simulink model "Ex_2"  (R2016b)
settings: Solver=ode3  StartTime=0.0  StopTime=10.0  RelTol=1e-3
libraries: Rayannik x3
settings Model: ExtModeTrigDuration=1000001  Creator=Alireza7  LastModifiedBy=Alireza7
settings RTWCC: SystemTargetFile=sldrt.tlc  TemplateMakefile=sldrt.tmf  Description=Simulink Desktop Real-Time  RTWCompilerOptimization=on
settings CodeAppCC: MaxIdLength=95
settings SimulinkDesktopRealTimeCC: TargetPreCompLibLocation=C:\Program Files\MATLAB\R2016b\toolbox\sldrt\lib\win64  SupportVariableSizeSignals=off

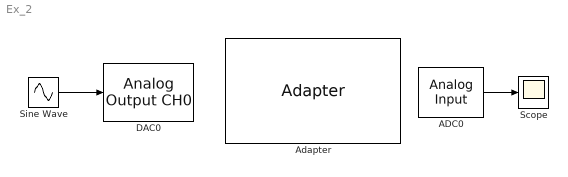
== system Ex_2 ==
  ADC0 : Rayannik/Analog Input  Priority=2  CH=0  vr=2.5  ou=Analog  inrr=-10 ~ +10
  Adapter : Rayannik/Adapter  SystemSampleTime=-1
      link override Packet Input1: SampleTime=Ts  MaxMissedTicks=1000000  ShowMissedTicks=off  YieldWhenWaiting=off  DrvName=Standard_Devices/Serial_Port  DrvAddress=3  DrvOptions=[9600 8 0 0 0 0 0 0]  PacketSize=33  DataTypes='33*uint8'  ShowReady=off  ShowError=off  PacketID=1  ByteOrder=1  ShowTimestamp=off
      link override Packet Output1: SampleTime=Ts  MaxMissedTicks=10000000  ShowMissedTicks=off  YieldWhenWaiting=off  DrvName=Standard_Devices/Serial_Port  DrvAddress=3  DrvOptions=[9600 8 0 0 0 0 0 0]  PacketSize=31  DataTypes='31*uint8'  ShowReady=off  ShowError=off  PacketID=1  ByteOrder=1  InitialValue=[]  FinalValue=[]
  DAC0 : Rayannik/Analog Output CH0  Priority=2  rfo=2.5  inpm=Analog  inr=-10 ~ +10
  Scope : Scope
  Sine Wave : Sin  Frequency=5  SampleTime=0
  wires:
  Sine Wave/1 -> DAC0/1
  ADC0/1 -> Scope/1
